simulink model "Ques7Ex5_AkankshaMurali"  (R2023b)
settings: Solver=VariableStepAuto  StartTime=0.0  StopTime=10.0  RelTol=1e-3
settings Model: Creator=akank  LastModifiedBy=akank

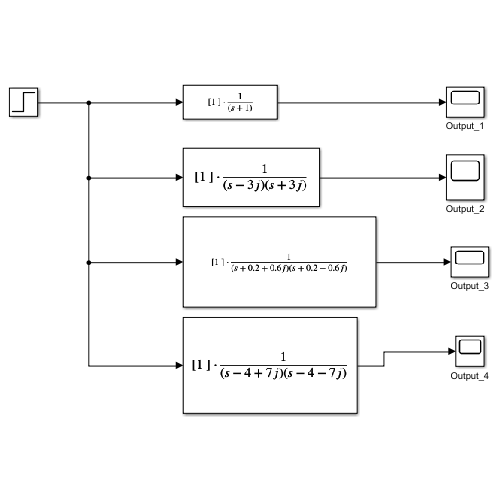
[thumbnail: Simulink's stored preview of the top-level diagram]
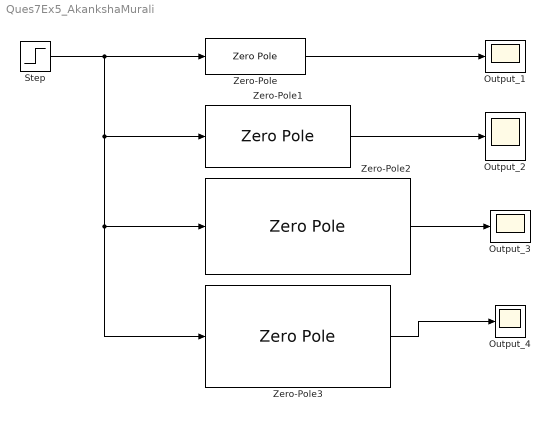
== system Ques7Ex5_AkankshaMurali ==
  Output_{1..4} (4 alike) : Scope
  Step : Step  Time=0  SampleTime=0
  Zero-Pole : ZeroPole  Zeros=[]  Poles=[-1]
  Zero-Pole1 : ZeroPole  Zeros=[]  Poles=[3j -3j]
  Zero-Pole2 : ZeroPole  Zeros=[]  Poles=[-0.2+0.6j -0.2-0.6j]
  Zero-Pole3 : ZeroPole  Zeros=[]  Poles=[4+7j 4-7j]
  wires:
  Zero-Pole1/1 -> Output_2/1
  Step/1 -> Zero-Pole3/1, Zero-Pole2/1, Zero-Pole1/1, Zero-Pole/1
  Zero-Pole3/1 -> Output_4/1
  Zero-Pole2/1 -> Output_3/1
  Zero-Pole/1 -> Output_1/1
